simulink model "Powertrain_model_21a"  (R2021a)
settings: Solver=VariableStepAuto  StartTime=0  StopTime=tspan  FixedStep=1  RelTol=1e-3
values from neighbouring files (symbols this model uses):
  bsfc_idle_CE = 31.7e03    (= 31700)    [Sim_script_conv.m]
  dailyloadl = Daily_Load_Hyb    [Sim_script_conv.m]
  DR = 5.213    [Sim_script_conv.m]
  MaxLimit = [700.510204081633	293.525179856115 ... (first row only)    [power_distribute_func.m]
  Trans_In = 24.086    [Sim_script_conv.m]
  tspan = 14400    [Sim_script_conv.m]
  w_CE_idle = 500    [Sim_script_conv.m]
undefined symbols (not defined in the file or in its folder): resT_conv_bollard, resT_conv_free, resT_conv_tow
libraries: pid_lib x1
settings Model: Creator=Sagar Singhal  LastModifiedBy=olsonsao
settings DataIOCC: SaveFormat=StructureWithTime
settings OptimizationCC: BlockReduction=off  BufferReuse=off
settings DebuggingCC: AlgebraicLoopMsg=none  UnconnectedInputMsg=none  UnconnectedOutputMsg=none  UnconnectedLineMsg=none

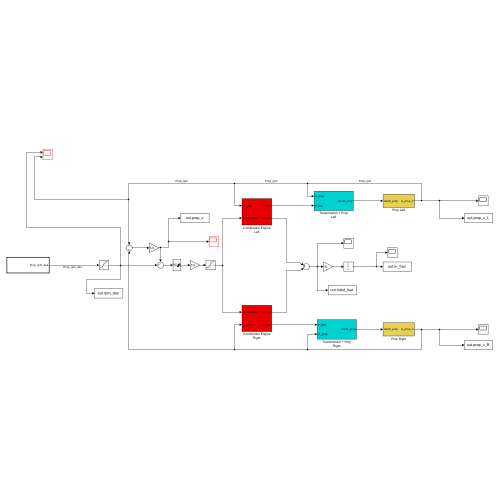
[thumbnail: Simulink's stored preview of the top-level diagram]
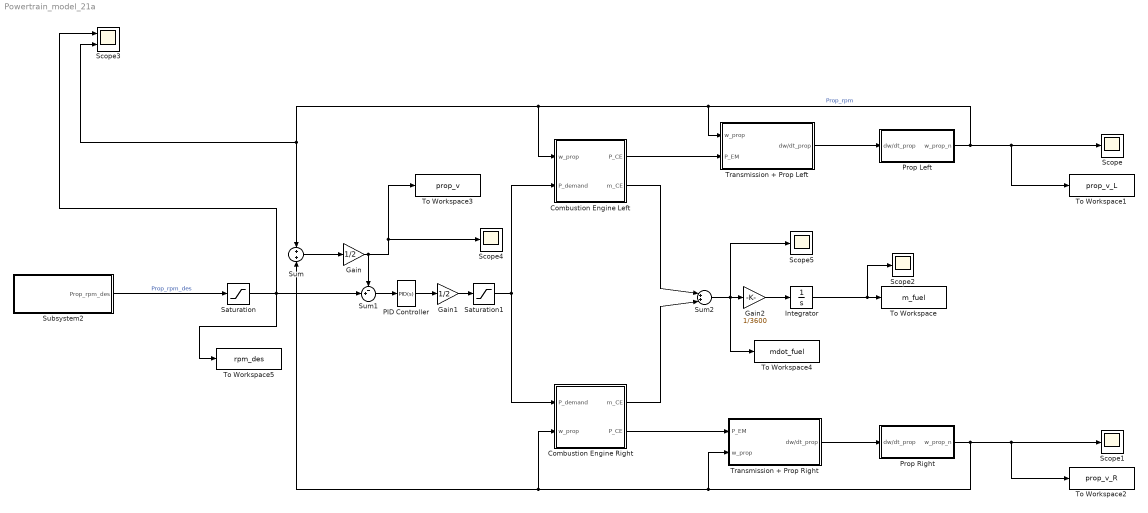
== system Powertrain_model_21a ==
  Combustion Engine Left : Subsystem  Tag=combustion engine
  Combustion Engine Right : Subsystem  Tag=combustion engine
  Gain : Gain  Gain=1/2
  Gain1 : Gain  Gain=1/2
  Gain2 : Gain  Gain=1/3600
  Integrator : Integrator
  PID Controller : pid_lib/PID Controller  Controller=PID  Form=Parallel  TimeDomain=Continuous-time  UseExternalTs=off  SampleTime=-1  IntegratorMethod=Forward Euler  FilterMethod=Forward Euler  ControllerParametersSource=internal  P=0.597253450179595  I=0.379410180722683  D=-1.14269148729982  UseFilter=on  N=0.349627806612909  TunerSelectOption=Transfer Function Based (PID Tuner App)  ZeroCross=off  InitialConditionSource=internal  InitialConditionForIntegrator=0  InitialConditionForFilter=0  DifferentiatorICPrevScaledInput=0  ExternalReset=none  TrackingMode=off  Kt=1  LimitOutput=on  SatLimitsSource=internal  UpperSaturationLimit=inf  LowerSaturationLimit=0  LinearizeAsGain=on  AntiWindupMode=none  Kb=1  POutMin=[]  POutMax=[]  IOutMin=[]  IOutMax=[]  DOutMin=[]  DOutMax=[]  NOutMin=[]  NOutMax=[]  SumOutMin=[]  SumOutMax=[]  SaturationOutMin=[]  SaturationOutMax=[]  PParamMin=[]  PParamMax=[]  IParamMin=[]  IParamMax=[]  DParamMin=[]  DParamMax=[]  NParamMin=[]  NParamMax=[]  KbParamMin=[]  KbParamMax=[]  KtParamMin=[]  KtParamMax=[]  KbOutMin=[]  KbOutMax=[]  KtOutMin=[]  KtOutMax=[]  IntegratorOutMin=[]  IntegratorOutMax=[]  FilterOutMin=[]  FilterOutMax=[]  SumI1OutMin=[]  SumI1OutMax=[]  SumI2OutMin=[]  SumI2OutMax=[]  SumI3OutMin=[]  SumI3OutMax=[]  SumI4OutMin=[]  SumI4OutMax=[]  SumDOutMin=[]  SumDOutMax=[]  DifferentiatorOutMin=[]  DifferentiatorOutMax=[]  FilterDiffOutCoefMin=[]  FilterDiffOutCoefMax=[]  ReciprocalOutMin=[]  ReciprocalOutMax=[]  SumDenOutMin=[]  SumDenOutMax=[]  SumNumOutMin=[]  SumNumOutMax=[]  DivideOutMin=[]  DivideOutMax=[]  UdiffTsProdOutMin=[]  UdiffTsProdOutMax=[]  NTsProdOutMin=[]  NTsProdOutMax=[]  UintegralTsProdOutMin=[]  UintegralTsProdOutMax=[]  UngainTsProdOutMin=[]  UngainTsProdOutMax=[]  IntegratorContinuousStateAttributes=''  IntegratorStateMustResolveToSignalObject=off  IntegratorRTWStateStorageClass=Auto  FilterContinuousStateAttributes=''  FilterStateMustResolveToSignalObject=off  FilterRTWStateStorageClass=Auto  ParallelPVariant=InternalParameters  IdealPVariant=Disabled  IVariant=InternalParameters  DVariant=InternalParameters  IntegratorVariant=Continuous  SatVariant=Enabled  AWVariant=Passthrough  PCopyVariant=Disabled  TRVariant=Disabled  FdbkBlocksVariant=Forward  IdealPFdbkVariant=Disabled  SatFdbkVariant=Disabled  DerivativeFilterVariant=ContFilter  NVariant=InternalParameters  NCopyVariant=Disabled  FilterICVariant=InternalICsFilter  IntegratorICVariant=InternalICs  ExternalResetVariant=Disabled  TRSumVariant=Passthrough  SumFdbkVariant=Disabled  SumVariant=Sum_PID  TsampFilterVariant=InternalTs  TsampNgainVariant=Passthrough  TsampIntegralVariant=Passthrough  ExternalSaturationOutDataTypeStr=Inherit: Same as second input
  Prop Left : Subsystem
  Prop Right : Subsystem
  Saturation : Saturate  UpperLimit=inf  LowerLimit=96
  Saturation1 : Saturate  UpperLimit=inf  LowerLimit=0
  Scope{,1..2,4..5} (5 alike) : Scope
  Scope3 : Scope  NumInputPorts=2
  Subsystem2 : Subsystem  TreatAsAtomicUnit=on
  Sum : Sum  Inputs=+|+
  Sum1 : Sum  Inputs=-+|
  Sum2 : Sum  Inputs=|++|
  To Workspace : ToWorkspace  VariableName=m_fuel  SampleTime=-1
      settings: Save2DSignal=2-D array (concatenate along first dimension)
  To Workspace1 : ToWorkspace  VariableName=prop_v_L  SampleTime=-1
      settings: Save2DSignal=2-D array (concatenate along first dimension)
  To Workspace2 : ToWorkspace  VariableName=prop_v_R  SampleTime=-1
      settings: Save2DSignal=2-D array (concatenate along first dimension)
  To Workspace3 : ToWorkspace  VariableName=prop_v  SampleTime=-1
      settings: Save2DSignal=2-D array (concatenate along first dimension)
  To Workspace4 : ToWorkspace  VariableName=mdot_fuel  SampleTime=-1
      settings: Save2DSignal=2-D array (concatenate along first dimension)
  To Workspace5 : ToWorkspace  VariableName=rpm_des  SampleTime=-1
      settings: Save2DSignal=2-D array (concatenate along first dimension)
  Transmission + Prop Left : Subsystem
  Transmission + Prop Right : Subsystem
  wires:
  Combustion Engine Left/1(P_CE) -> Transmission + Prop Left/2(P_EM)
  Transmission + Prop Left/1(dw/dt_prop) -> Prop Left/1(dw/dt_prop)
  Combustion Engine Left/2(m_CE) -> Sum2/1
  Prop Left/1(w_prop_n) -> To Workspace1/1, Scope/1, Transmission + Prop Left/1(w_prop), Combustion Engine Left/1(w_prop), Scope3/2, Sum/1  "Prop_rpm"
  Prop Right/1(w_prop_n) -> Transmission + Prop Right/2(w_prop), Combustion Engine Right/2(w_prop), Sum/2, To Workspace2/1, Scope1/1
  Transmission + Prop Right/1(dw/dt_prop) -> Prop Right/1(dw/dt_prop)
  Combustion Engine Right/1(m_CE) -> Sum2/2
  Sum/1 -> Gain/1
  Saturation/1 -> To Workspace5/1, Sum1/2, Scope3/1
  Subsystem2/1(Prop_rpm_des) -> Saturation/1  "Prop_rpm_des"
  Gain/1 -> To Workspace3/1, Scope4/1, Sum1/1
  Sum1/1 -> PID Controller/1
  PID Controller/1 -> Gain1/1
  Gain1/1 -> Saturation1/1
  Saturation1/1 -> Combustion Engine Left/2(P_demand), Combustion Engine Right/1(P_demand)
  Sum2/1 -> To Workspace4/1, Scope5/1, Gain2/1
  Integrator/1 -> Scope2/1, To Workspace/1
  Gain2/1 -> Integrator/1
  Combustion Engine Right/2(P_CE) -> Transmission + Prop Right/1(P_EM)

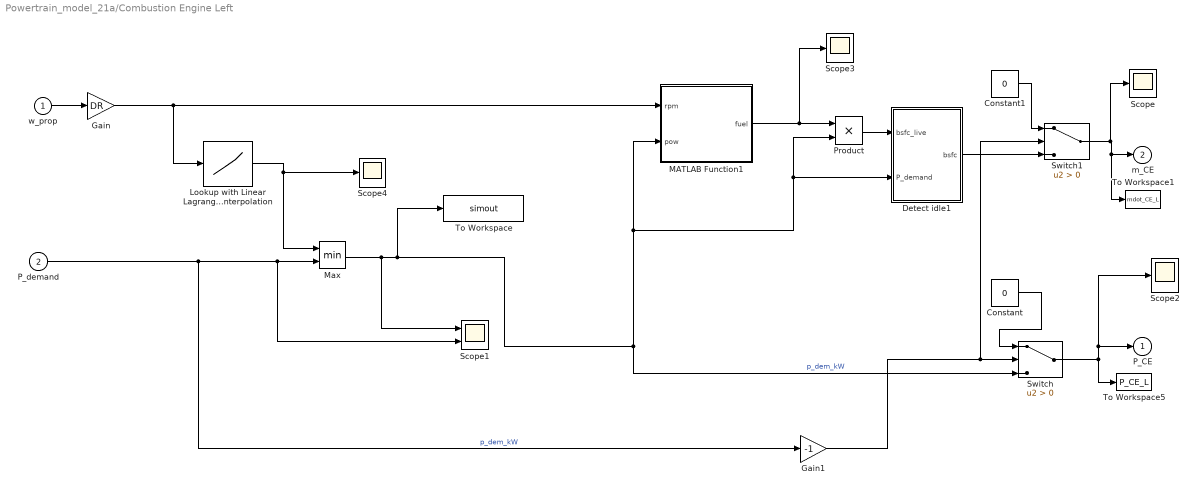
== system Powertrain_model_21a/Combustion Engine Left ==
  w_prop : Inport
  P_demand : Inport  Port=2
  Constant : Constant  Value=0
  Constant1 : Constant  Value=0
  Detect idle1 : Subsystem
  Gain : Gain  Gain=DR
  Gain1 : Gain  Gain=-1
  Lookup with Linear Lagrange Interpolation : Lookup_n-D  NumberOfTableDimensions=1  BreakpointsForDimension1=MaxLimit.('RPM')  Table=MaxLimit.('Pow_kW_')  InternalRulePriority=Speed  RndMeth=Simplest  InputSameDT=on
  MATLAB Function1 : MATLAB Function  TreatAsAtomicUnit=on
  Max : MinMax  Inputs=2
  Product : Product
  Scope{,2..4} (4 alike) : Scope
  Scope1 : Scope  NumInputPorts=2
  Switch : Switch  Criteria=u2 > Threshold
  Switch1 : Switch  Criteria=u2 > Threshold
  To Workspace : ToWorkspace  VariableName=simout  SampleTime=-1
      settings: Save2DSignal=2-D array (concatenate along first dimension)
  To Workspace1 : ToWorkspace  VariableName=mdot_CE_L  SampleTime=-1
      settings: Save2DSignal=2-D array (concatenate along first dimension)
  To Workspace5 : ToWorkspace  VariableName=P_CE_L  SampleTime=-1
      settings: Save2DSignal=2-D array (concatenate along first dimension)
  P_CE : Outport  InitialOutput=0
  m_CE : Outport  Port=2  InitialOutput=0
  wires:
  w_prop/1 -> Gain/1
  Lookup with Linear Lagrange Interpolation/1 -> Max/1, Scope4/1
  MATLAB Function1/1(fuel) -> Scope3/1, Product/1
  Gain/1 -> Lookup with Linear Lagrange Interpolation/1, MATLAB Function1/1(rpm)
  Max/1 -> Scope1/1, To Workspace/1, Switch/3, Product/2, Detect idle1/2(P_demand), MATLAB Function1/2(pow)  "p_dem_kW"
  P_demand/1 -> Gain1/1, Scope1/2, Max/2  "p_dem_kW"
  Product/1 -> Detect idle1/1(bsfc_live)
  Gain1/1 -> Switch1/2, Switch/2
  Constant/1 -> Switch/1
  Switch/1 -> Scope2/1, P_CE/1, To Workspace5/1
  Constant1/1 -> Switch1/1
  Detect idle1/1(bsfc) -> Switch1/3
  Switch1/1 -> Scope/1, To Workspace1/1, m_CE/1

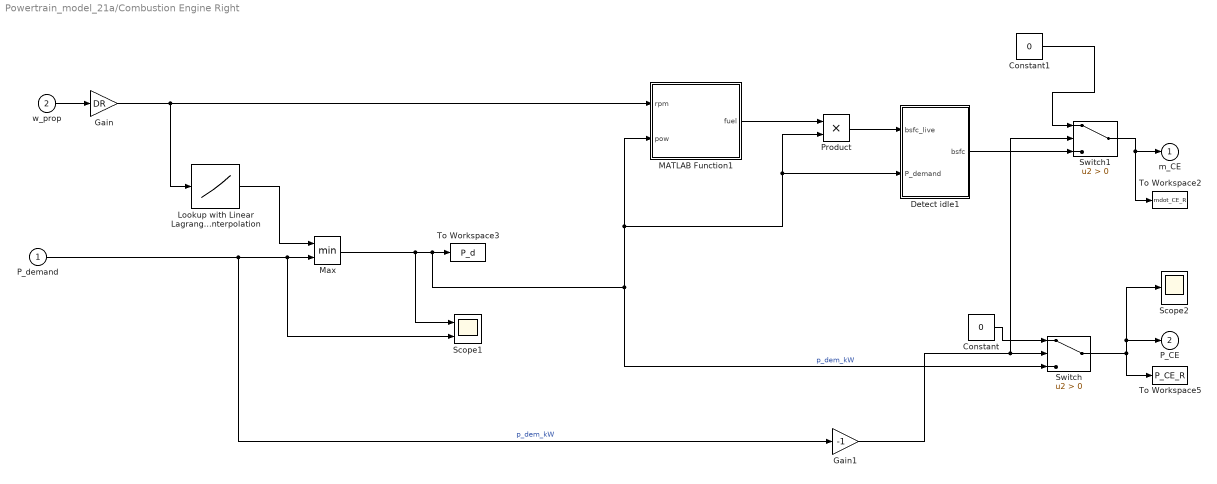
== system Powertrain_model_21a/Combustion Engine Right ==
  P_demand : Inport
  w_prop : Inport  Port=2
  Constant : Constant  Value=0
  Constant1 : Constant  Value=0
  Detect idle1 : Subsystem
  Gain : Gain  Gain=DR
  Gain1 : Gain  Gain=-1
  Lookup with Linear Lagrange Interpolation : Lookup_n-D  NumberOfTableDimensions=1  BreakpointsForDimension1=MaxLimit.('RPM')  Table=MaxLimit.('Pow_kW_')  InternalRulePriority=Speed  RndMeth=Simplest  InputSameDT=on
  MATLAB Function1 : MATLAB Function  TreatAsAtomicUnit=on
  Max : MinMax  Inputs=2
  Product : Product
  Scope1 : Scope  NumInputPorts=2
  Scope2 : Scope
  Switch : Switch  Criteria=u2 > Threshold
  Switch1 : Switch  Criteria=u2 > Threshold
  To Workspace2 : ToWorkspace  VariableName=mdot_CE_R  SampleTime=-1
      settings: Save2DSignal=2-D array (concatenate along first dimension)
  To Workspace3 : ToWorkspace  VariableName=P_d  SampleTime=-1
      settings: Save2DSignal=2-D array (concatenate along first dimension)
  To Workspace5 : ToWorkspace  VariableName=P_CE_R  SampleTime=-1
      settings: Save2DSignal=2-D array (concatenate along first dimension)
  m_CE : Outport  InitialOutput=0
  P_CE : Outport  Port=2  InitialOutput=0
  wires:
  w_prop/1 -> Gain/1
  Lookup with Linear Lagrange Interpolation/1 -> Max/1
  MATLAB Function1/1(fuel) -> Product/1
  Gain/1 -> Lookup with Linear Lagrange Interpolation/1, MATLAB Function1/1(rpm)
  Product/1 -> Detect idle1/1(bsfc_live)
  Max/1 -> Scope1/1, Switch/3, Detect idle1/2(P_demand), Product/2, MATLAB Function1/2(pow), To Workspace3/1  "p_dem_kW"
  Detect idle1/1(bsfc) -> Switch1/3
  Constant/1 -> Switch/1
  Gain1/1 -> Switch1/2, Switch/2
  P_demand/1 -> Gain1/1, Scope1/2, Max/2  "p_dem_kW"
  Switch/1 -> Scope2/1, P_CE/1, To Workspace5/1
  Constant1/1 -> Switch1/1
  Switch1/1 -> To Workspace2/1, m_CE/1

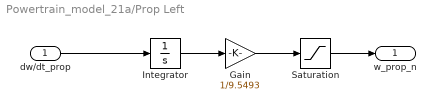
== system Powertrain_model_21a/Prop Left ==
  dw/dt_prop : Inport
  Gain : Gain  Gain=1/9.5493
  Integrator : Integrator  InitialCondition=200  LimitOutput=on  LowerSaturationLimit=0
  Saturation : Saturate  UpperLimit=inf  LowerLimit=w_CE_idle/DR
  w_prop_n : Outport
  wires:
  dw/dt_prop/1 -> Integrator/1
  Integrator/1 -> Gain/1
  Saturation/1 -> w_prop_n/1
  Gain/1 -> Saturation/1

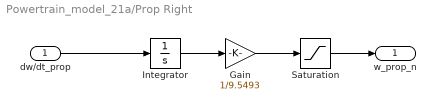
== system Powertrain_model_21a/Prop Right ==
  dw/dt_prop : Inport
  Gain : Gain  Gain=1/9.5493
  Integrator : Integrator  InitialCondition=200  LimitOutput=on  LowerSaturationLimit=0
  Saturation : Saturate  UpperLimit=inf  LowerLimit=0
  w_prop_n : Outport
  wires:
  dw/dt_prop/1 -> Integrator/1
  Integrator/1 -> Gain/1
  Saturation/1 -> w_prop_n/1
  Gain/1 -> Saturation/1

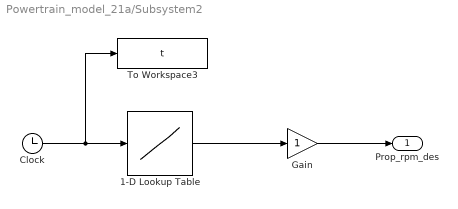
== system Powertrain_model_21a/Subsystem2 ==
  1-D Lookup Table : Lookup_n-D  NumberOfTableDimensions=1  BreakpointsForDimension1=[1:tspan]  Table=dailyloadl.('rpm')  InternalRulePriority=Speed  RndMeth=Simplest  InputSameDT=on
  Clock : Clock
  Gain : Gain
  To Workspace3 : ToWorkspace  VariableName=t  SampleTime=-1
      settings: Save2DSignal=2-D array (concatenate along first dimension)
  Prop_rpm_des : Outport
  wires:
  Clock/1 -> To Workspace3/1, 1-D Lookup Table/1
  1-D Lookup Table/1 -> Gain/1
  Gain/1 -> Prop_rpm_des/1

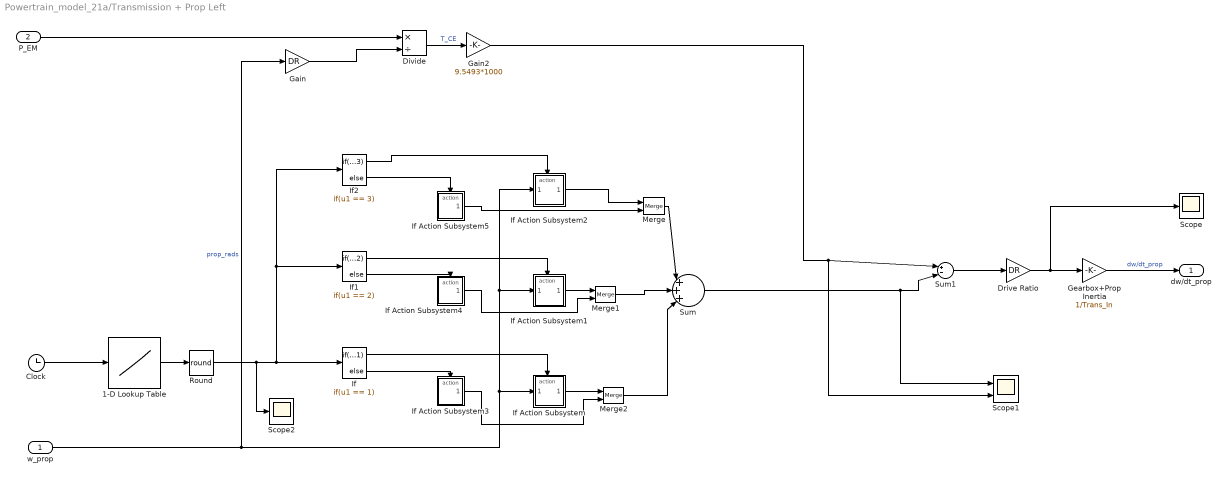
== system Powertrain_model_21a/Transmission + Prop Left ==
  w_prop : Inport
  P_EM : Inport  Port=2
  1-D Lookup Table : Lookup_n-D  NumberOfTableDimensions=1  BreakpointsForDimension1=[1:tspan]  Table=dailyloadl.('mode')  InternalRulePriority=Speed  RndMeth=Simplest  InputSameDT=on
  Clock : Clock
  Divide : Product  Inputs=*/
  Drive Ratio : Gain  Gain=DR
  Gain : Gain  Gain=DR
  Gain2 : Gain  Gain=9.5493*1000
  Gearbox+Prop Inertia : Gain  Gain=1/Trans_In
  If : If  IfExpression=u1 == 1
  If Action Subsystem : Subsystem  TreatAsAtomicUnit=on
  If Action Subsystem1 : Subsystem  TreatAsAtomicUnit=on
  If Action Subsystem2 : Subsystem  TreatAsAtomicUnit=on
  If Action Subsystem3 : Subsystem  TreatAsAtomicUnit=on
  If Action Subsystem4 : Subsystem  TreatAsAtomicUnit=on
  If Action Subsystem5 : Subsystem  TreatAsAtomicUnit=on
  If1 : If  IfExpression=u1 == 2
  If2 : If  IfExpression=u1 == 3
  Merge : Merge
  Merge1 : Merge
  Merge2 : Merge
  Round : Rounding  Operator=round
  Scope : Scope
  Scope1 : Scope  NumInputPorts=2
  Scope2 : Scope
  Sum : Sum  Inputs=|+++|
  Sum1 : Sum  Inputs=|+-|
  dw/dt_prop : Outport
  wires:
  P_EM/1 -> Divide/1
  Gearbox+Prop Inertia/1 -> dw/dt_prop/1  "dw/dt_prop"
  Sum1/1 -> Drive Ratio/1
  Divide/1 -> Gain2/1  "T_CE"
  Gain2/1 -> Scope1/2, Sum1/1
  w_prop/1 -> If Action Subsystem2/1(w_prop), If Action Subsystem1/1(w_prop), If Action Subsystem/1(w_prop), Gain/1  "prop_rads"
  1-D Lookup Table/1 -> Round/1
  Clock/1 -> 1-D Lookup Table/1
  If/1 -> If Action Subsystem/Action
  If/2 -> If Action Subsystem3/Action
  If1/1 -> If Action Subsystem1/Action
  If2/1 -> If Action Subsystem2/Action
  If2/2 -> If Action Subsystem5/Action
  If1/2 -> If Action Subsystem4/Action
  If Action Subsystem2/1(Out1) -> Merge/1
  If Action Subsystem5/1(Out1) -> Merge/2
  If Action Subsystem1/1(Out1) -> Merge1/1
  Round/1 -> Scope2/1, If1/1, If2/1, If/1
  Merge/1 -> Sum/1
  If Action Subsystem4/1(Out1) -> Merge1/2
  If Action Subsystem/1(Out1) -> Merge2/1
  If Action Subsystem3/1(Out1) -> Merge2/2
  Merge1/1 -> Sum/2
  Merge2/1 -> Sum/3
  Drive Ratio/1 -> Gearbox+Prop Inertia/1, Scope/1
  Sum/1 -> Scope1/1, Sum1/2
  Gain/1 -> Divide/2

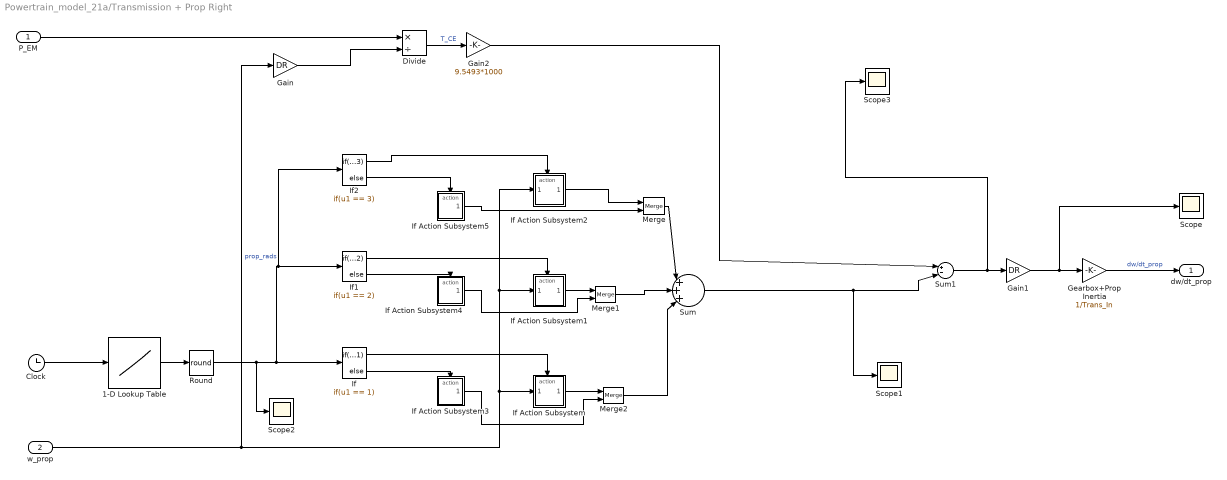
== system Powertrain_model_21a/Transmission + Prop Right ==
  P_EM : Inport
  w_prop : Inport  Port=2
  1-D Lookup Table : Lookup_n-D  NumberOfTableDimensions=1  BreakpointsForDimension1=[1:tspan]  Table=dailyloadl.('mode')  InternalRulePriority=Speed  RndMeth=Simplest  InputSameDT=on
  Clock : Clock
  Divide : Product  Inputs=*/
  Gain : Gain  Gain=DR
  Gain1 : Gain  Gain=DR
  Gain2 : Gain  Gain=9.5493*1000
  Gearbox+Prop Inertia : Gain  Gain=1/Trans_In
  If : If  IfExpression=u1 == 1
  If Action Subsystem : Subsystem  TreatAsAtomicUnit=on
  If Action Subsystem1 : Subsystem  TreatAsAtomicUnit=on
  If Action Subsystem2 : Subsystem  TreatAsAtomicUnit=on
  If Action Subsystem3 : Subsystem  TreatAsAtomicUnit=on
  If Action Subsystem4 : Subsystem  TreatAsAtomicUnit=on
  If Action Subsystem5 : Subsystem  TreatAsAtomicUnit=on
  If1 : If  IfExpression=u1 == 2
  If2 : If  IfExpression=u1 == 3
  Merge : Merge
  Merge1 : Merge
  Merge2 : Merge
  Round : Rounding  Operator=round
  Scope{,1..3} (4 alike) : Scope
  Sum : Sum  Inputs=|+++|
  Sum1 : Sum  Inputs=|+-|
  dw/dt_prop : Outport
  wires:
  P_EM/1 -> Divide/1
  Gearbox+Prop Inertia/1 -> dw/dt_prop/1  "dw/dt_prop"
  Sum1/1 -> Scope3/1, Gain1/1
  Divide/1 -> Gain2/1  "T_CE"
  Gain2/1 -> Sum1/1
  w_prop/1 -> If Action Subsystem2/1(w_prop), If Action Subsystem1/1(w_prop), If Action Subsystem/1(w_prop), Gain/1  "prop_rads"
  1-D Lookup Table/1 -> Round/1
  Clock/1 -> 1-D Lookup Table/1
  If/1 -> If Action Subsystem/Action
  If/2 -> If Action Subsystem3/Action
  If1/1 -> If Action Subsystem1/Action
  If2/1 -> If Action Subsystem2/Action
  If2/2 -> If Action Subsystem5/Action
  If1/2 -> If Action Subsystem4/Action
  If Action Subsystem2/1(Out1) -> Merge/1
  If Action Subsystem5/1(Out1) -> Merge/2
  If Action Subsystem1/1(Out1) -> Merge1/1
  Round/1 -> Scope2/1, If2/1, If1/1, If/1
  Merge/1 -> Sum/1
  If Action Subsystem4/1(Out1) -> Merge1/2
  If Action Subsystem/1(Out1) -> Merge2/1
  If Action Subsystem3/1(Out1) -> Merge2/2
  Merge1/1 -> Sum/2
  Merge2/1 -> Sum/3
  Gain1/1 -> Gearbox+Prop Inertia/1, Scope/1
  Sum/1 -> Sum1/2, Scope1/1
  Gain/1 -> Divide/2

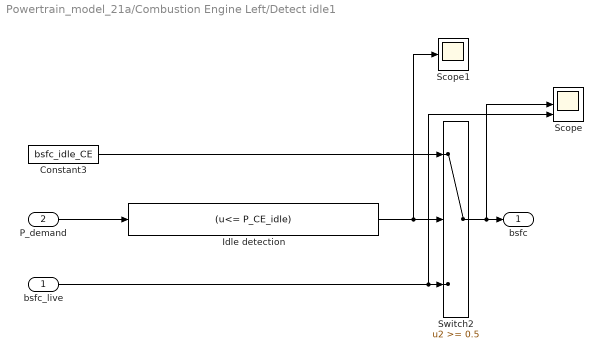
== system Powertrain_model_21a/Combustion Engine Left/Detect idle1 ==
  bsfc_live : Inport
  P_demand : Inport  Port=2
  Constant3 : Constant  Value=bsfc_idle_CE
  Idle detection : Fcn  Expr=(u<= P_CE_idle)
  Scope : Scope  NumInputPorts=3
  Scope1 : Scope
  Switch2 : Switch  Threshold=0.5  SaturateOnIntegerOverflow=on  InputSameDT=on
  bsfc : Outport  InitialOutput=0
  wires:
  P_demand/1 -> Idle detection/1
  Idle detection/1 -> Scope1/1, Switch2/2
  bsfc_live/1 -> Scope/3, Switch2/3
  Switch2/1 -> Scope/2, bsfc/1
  Constant3/1 -> Switch2/1

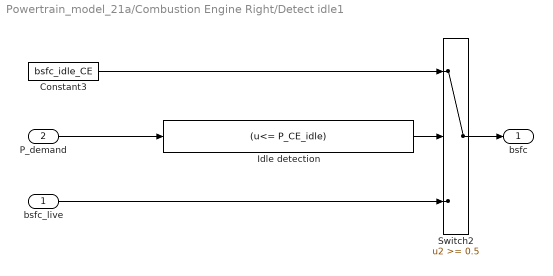
== system Powertrain_model_21a/Combustion Engine Right/Detect idle1 ==
  bsfc_live : Inport
  P_demand : Inport  Port=2
  Constant3 : Constant  Value=bsfc_idle_CE
  Idle detection : Fcn  Expr=(u<= P_CE_idle)
  Switch2 : Switch  Threshold=0.5  SaturateOnIntegerOverflow=on  InputSameDT=on
  bsfc : Outport  InitialOutput=0
  wires:
  P_demand/1 -> Idle detection/1
  Idle detection/1 -> Switch2/2
  bsfc_live/1 -> Switch2/3
  Switch2/1 -> bsfc/1
  Constant3/1 -> Switch2/1

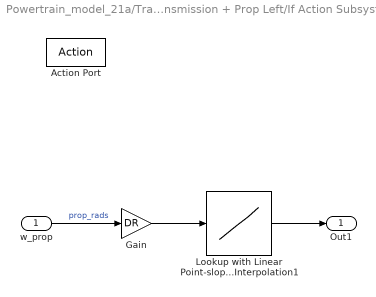
== system Powertrain_model_21a/Transmission + Prop Left/If Action Subsystem ==
  w_prop : Inport
  Action Port : ActionPort  ActionPortLabel=if(u1 == 1)
  Gain : Gain  Gain=DR
  Lookup with Linear Point-slope Interpolation1 : Lookup_n-D  NumberOfTableDimensions=1  BreakpointsForDimension1=resT_conv_free.('rpm')  Table=resT_conv_free.('resT')  InternalRulePriority=Speed  RndMeth=Simplest  InputSameDT=on
  Out1 : Outport
  wires:
  Lookup with Linear Point-slope Interpolation1/1 -> Out1/1
  w_prop/1 -> Gain/1  "prop_rads"
  Gain/1 -> Lookup with Linear Point-slope Interpolation1/1

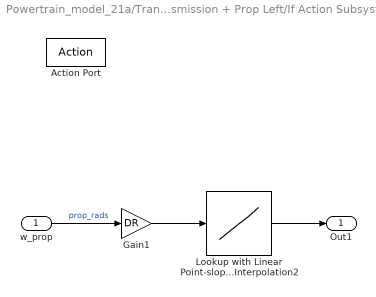
== system Powertrain_model_21a/Transmission + Prop Left/If Action Subsystem1 ==
  w_prop : Inport
  Action Port : ActionPort  ActionPortLabel=if(u1 == 2)
  Gain1 : Gain  Gain=DR
  Lookup with Linear Point-slope Interpolation2 : Lookup_n-D  NumberOfTableDimensions=1  BreakpointsForDimension1=resT_conv_tow.('rpm')  Table=resT_conv_tow.('resT')  InternalRulePriority=Speed  RndMeth=Simplest  InputSameDT=on
  Out1 : Outport
  wires:
  Lookup with Linear Point-slope Interpolation2/1 -> Out1/1
  Gain1/1 -> Lookup with Linear Point-slope Interpolation2/1
  w_prop/1 -> Gain1/1  "prop_rads"

== system Powertrain_model_21a/Transmission + Prop Left/If Action Subsystem2 ==
  w_prop : Inport
  Action Port : ActionPort  ActionPortLabel=if(u1 == 3)
  Gain3 : Gain  Gain=DR
  Lookup with Linear Point-slope Interpolation3 : Lookup_n-D  NumberOfTableDimensions=1  BreakpointsForDimension1=resT_conv_bollard.('rpm')  Table=resT_conv_bollard.('resT')  InternalRulePriority=Speed  RndMeth=Simplest  InputSameDT=on
  Out1 : Outport
  wires:
  Lookup with Linear Point-slope Interpolation3/1 -> Out1/1
  Gain3/1 -> Lookup with Linear Point-slope Interpolation3/1
  w_prop/1 -> Gain3/1  "prop_rads"

== system Powertrain_model_21a/Transmission + Prop Left/If Action Subsystem3 ==
  Action Port : ActionPort  ActionPortLabel=else
  Constant : Constant  Value=0
  Out1 : Outport
  wires:
  Constant/1 -> Out1/1

== system Powertrain_model_21a/Transmission + Prop Left/If Action Subsystem4 ==
  Action Port : ActionPort  ActionPortLabel=else
  Constant : Constant  Value=0
  Out1 : Outport
  wires:
  Constant/1 -> Out1/1

== system Powertrain_model_21a/Transmission + Prop Left/If Action Subsystem5 ==
  Action Port : ActionPort  ActionPortLabel=else
  Constant : Constant  Value=0
  Out1 : Outport
  wires:
  Constant/1 -> Out1/1

== system Powertrain_model_21a/Transmission + Prop Right/If Action Subsystem ==
  w_prop : Inport
  Action Port : ActionPort  ActionPortLabel=if(u1 == 1)
  Gain : Gain  Gain=DR
  Lookup with Linear Point-slope Interpolation1 : Lookup_n-D  NumberOfTableDimensions=1  BreakpointsForDimension1=resT_conv_free.('rpm')  Table=resT_conv_free.('resT')  InternalRulePriority=Speed  RndMeth=Simplest  InputSameDT=on
  Out1 : Outport
  wires:
  Lookup with Linear Point-slope Interpolation1/1 -> Out1/1
  w_prop/1 -> Gain/1  "prop_rads"
  Gain/1 -> Lookup with Linear Point-slope Interpolation1/1

== system Powertrain_model_21a/Transmission + Prop Right/If Action Subsystem1 ==
  w_prop : Inport
  Action Port : ActionPort  ActionPortLabel=if(u1 == 2)
  Gain1 : Gain  Gain=DR
  Lookup with Linear Point-slope Interpolation2 : Lookup_n-D  NumberOfTableDimensions=1  BreakpointsForDimension1=resT_conv_tow.('rpm')  Table=resT_conv_tow.('resT')  InternalRulePriority=Speed  RndMeth=Simplest  InputSameDT=on
  Out1 : Outport
  wires:
  Lookup with Linear Point-slope Interpolation2/1 -> Out1/1
  Gain1/1 -> Lookup with Linear Point-slope Interpolation2/1
  w_prop/1 -> Gain1/1  "prop_rads"

== system Powertrain_model_21a/Transmission + Prop Right/If Action Subsystem2 ==
  w_prop : Inport
  Action Port : ActionPort  ActionPortLabel=if(u1 == 3)
  Gain3 : Gain  Gain=DR
  Lookup with Linear Point-slope Interpolation3 : Lookup_n-D  NumberOfTableDimensions=1  BreakpointsForDimension1=resT_conv_bollard.('rpm')  Table=resT_conv_bollard.('resT')  InternalRulePriority=Speed  RndMeth=Simplest  InputSameDT=on
  Out1 : Outport
  wires:
  Lookup with Linear Point-slope Interpolation3/1 -> Out1/1
  Gain3/1 -> Lookup with Linear Point-slope Interpolation3/1
  w_prop/1 -> Gain3/1  "prop_rads"

== system Powertrain_model_21a/Transmission + Prop Right/If Action Subsystem3 ==
  Action Port : ActionPort  ActionPortLabel=else
  Constant : Constant  Value=0
  Out1 : Outport
  wires:
  Constant/1 -> Out1/1

== system Powertrain_model_21a/Transmission + Prop Right/If Action Subsystem4 ==
  Action Port : ActionPort  ActionPortLabel=else
  Constant : Constant  Value=0
  Out1 : Outport
  wires:
  Constant/1 -> Out1/1

== system Powertrain_model_21a/Transmission + Prop Right/If Action Subsystem5 ==
  Action Port : ActionPort  ActionPortLabel=else
  Constant : Constant  Value=0
  Out1 : Outport
  wires:
  Constant/1 -> Out1/1

== matlab function Powertrain_model_21a/Combustion Engine Right/MATLAB Function1 ==
  data: rpm input; fuel output; pow input
function fuel = bsfc_map(rpm,pow)

    fuel = fuel_con_map(rpm,pow);
end

== matlab function Powertrain_model_21a/Combustion Engine Left/MATLAB Function1 ==
  data: rpm input; fuel output; pow input
function fuel = bsfc_map(rpm,pow)

    fuel = fuel_con_map(rpm,pow);
end
